simulink library "rocket_angular_flight_library"  (R2014a)
settings: Solver=ode45  StartTime=0.0  StopTime=10.0  RelTol=1e-3
undefined symbols (not defined in the file or in its folder): area_rocket_planform, cog_motor, d_nose_tip_to_fins, d_nose_tip_to_nozzle, diameter_outer, dry_rocket_mass, F, factstruct, fin_center_distance, fin_root_chord, fin_tip_chord, fins_count, height_fins, height_nose_cone, length_motor, Light, mass_flow_rate, MIL, motorburntime
libraries: rocket_angular_flight_library x10, rocket_dynamic_data_library x3, simulink x2, aerolibadyn x2, aerolibbdyn x2, aerolib6dof2 x1, aerolibasang x1, aerolibwind2 x1
settings Model: Creator=scorpii  LastModifiedBy=scorpii

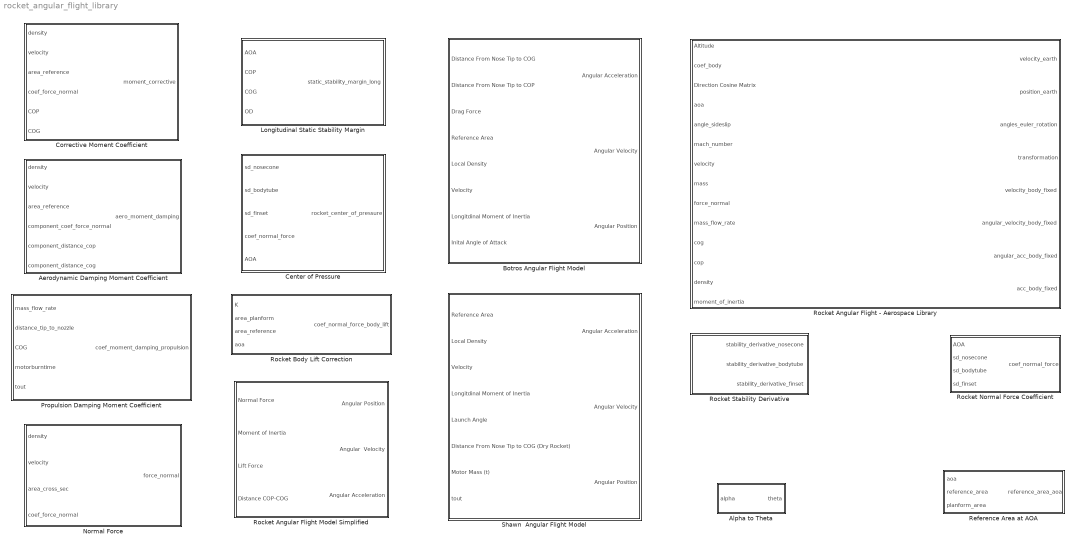
== system rocket_angular_flight_library ==
  Aerodynamic Damping Moment Coefficient : Subsystem  AncestorBlock=rocket_angular_flight_library/Corrective Moment Coefficient
  Alpha to Theta : Subsystem
  Botros Angular Flight Model : Subsystem
  Center of Pressure : Subsystem
  Corrective Moment Coefficient : Subsystem
  Longitudinal Static Stability Margin : Subsystem
  Normal Force : Subsystem
  Propulsion Damping Moment Coefficient : Subsystem
  Reference Area at AOA : Subsystem
  Rocket Angular Flight - Aerospace Library : Subsystem
  Rocket Angular Flight Model Simplified : Subsystem  AncestorBlock=rocket_vertical_flight_library/Rocket Vertical Flight Model
  Rocket Body Lift Correction : Subsystem
  Rocket Normal Force Coefficient : Subsystem
  Rocket Stability Derivative : Subsystem  TreatAsAtomicUnit=on
  Shawn  Angular Flight Model : Subsystem  AncestorBlock=rocket_angular_flight_library/Angular Flight Model

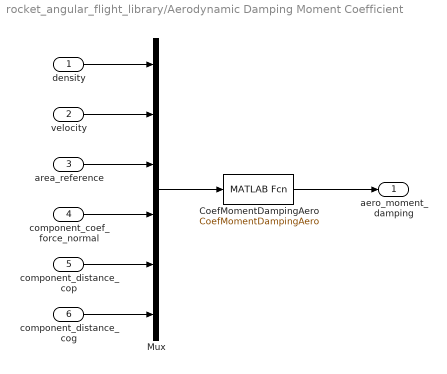
== system rocket_angular_flight_library/Aerodynamic Damping Moment Coefficient ==
  density : Inport
  velocity : Inport  Port=2
  area_reference : Inport  Port=3
  component_coef_force_normal : Inport  Port=4
  component_distance_cop : Inport  Port=5
  component_distance_cog : Inport  Port=6
  CoefMomentDampingAero : MATLABFcn  MATLABFcn=CoefMomentDampingAero
  Mux : Mux  Inputs=6
  aero_moment_damping : Outport
  wires:
  density/1 -> Mux/1
  velocity/1 -> Mux/2
  area_reference/1 -> Mux/3
  component_coef_force_normal/1 -> Mux/4
  component_distance_cop/1 -> Mux/5
  component_distance_cog/1 -> Mux/6
  Mux/1 -> CoefMomentDampingAero/1
  CoefMomentDampingAero/1 -> aero_moment_damping/1

== system rocket_angular_flight_library/Alpha to Theta ==
  alpha : Inport
  Abs : Abs
  Constant : Constant  Value=pi/2
  Subtract : Sum  Inputs=+-
  theta : Outport
  wires:
  Constant/1 -> Subtract/1
  alpha/1 -> Subtract/2
  Subtract/1 -> Abs/1
  Abs/1 -> theta/1

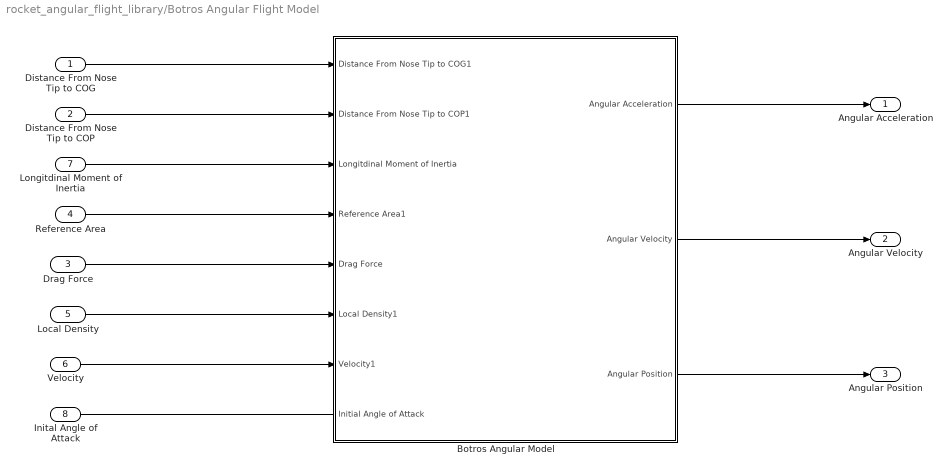
== system rocket_angular_flight_library/Botros Angular Flight Model ==
  Distance From Nose Tip to COG : Inport
  Distance From Nose Tip to COP : Inport  Port=2
  Drag Force : Inport  Port=3
  Reference Area : Inport  Port=4
  Local Density : Inport  Port=5
  Velocity : Inport  Port=6
  "Longitdinal Moment of Inertia " : Inport  Port=7
  Inital Angle of Attack : Inport  Port=8
  Botros Angular Model : Subsystem
  Angular Acceleration : Outport
  Angular Velocity : Outport  Port=2
  Angular Position : Outport  Port=3
  wires:
  Distance From Nose Tip to COP/1 -> Botros Angular Model/2(Distance From Nose Tip to COP1)
  Drag Force/1 -> Botros Angular Model/5(Drag Force)
  Velocity/1 -> Botros Angular Model/7(Velocity1)
  Local Density/1 -> Botros Angular Model/6(Local Density1)
  Reference Area/1 -> Botros Angular Model/4(Reference Area1)
  Botros Angular Model/3(Angular Position) -> Angular Position/1
  Botros Angular Model/1(Angular Acceleration) -> Angular Acceleration/1
  Botros Angular Model/2(Angular Velocity) -> Angular Velocity/1
  "Longitdinal Moment of Inertia "/1 -> Botros Angular Model/3(Longitdinal Moment of Inertia)
  Inital Angle of Attack/1 -> ?
  Distance From Nose Tip to COG/1 -> Botros Angular Model/1(Distance From Nose Tip to COG1)

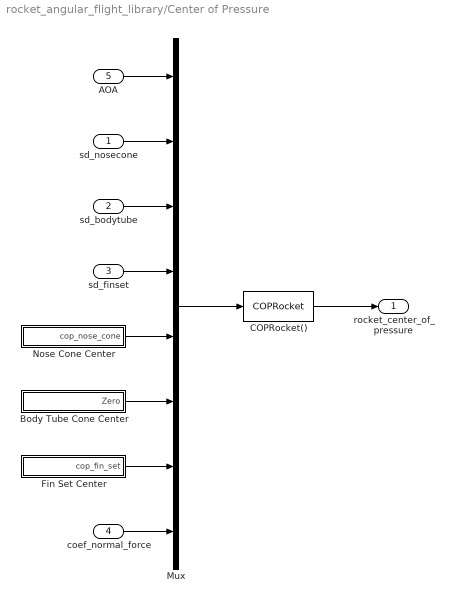
== system rocket_angular_flight_library/Center of Pressure ==
  sd_nosecone : Inport
  sd_bodytube : Inport  Port=2
  sd_finset : Inport  Port=3
  coef_normal_force : Inport  Port=4
  AOA : Inport  Port=5
  Body Tube Cone Center : Subsystem  AncestorBlock=rocket_angular_flight_library/Center of Pressure/Nose Cone Center
  COPRocket() : MATLABFcn  MATLABFcn=COPRocket
  Fin Set Center : Subsystem
  Mux : Mux  Inputs=8
  Nose Cone Center : Subsystem  AncestorBlock=rocket_angular_flight_library/Center of Pressure/Nose Cone Center
  rocket_center_of_pressure : Outport
  wires:
  Mux/1 -> COPRocket()/1
  COPRocket()/1 -> rocket_center_of_pressure/1
  AOA/1 -> Mux/1
  coef_normal_force/1 -> Mux/8
  sd_nosecone/1 -> Mux/2
  sd_bodytube/1 -> Mux/3
  sd_finset/1 -> Mux/4
  Nose Cone Center/1(cop_nose_cone) -> Mux/5
  Fin Set Center/1(cop_fin_set) -> Mux/7
  Body Tube Cone Center/1(Zero) -> Mux/6

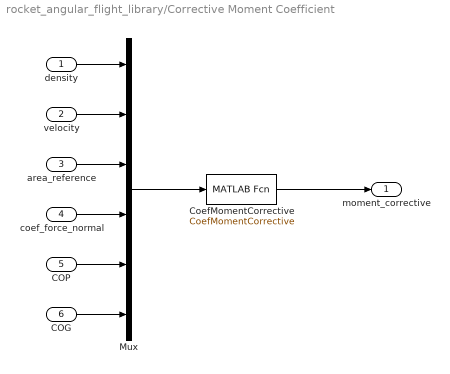
== system rocket_angular_flight_library/Corrective Moment Coefficient ==
  density : Inport
  velocity : Inport  Port=2
  area_reference : Inport  Port=3
  coef_force_normal : Inport  Port=4
  COP : Inport  Port=5
  COG : Inport  Port=6
  CoefMomentCorrective : MATLABFcn  MATLABFcn=CoefMomentCorrective
  Mux : Mux  Inputs=6
  moment_corrective : Outport
  wires:
  density/1 -> Mux/1
  velocity/1 -> Mux/2
  area_reference/1 -> Mux/3
  coef_force_normal/1 -> Mux/4
  COP/1 -> Mux/5
  COG/1 -> Mux/6
  Mux/1 -> CoefMomentCorrective/1
  CoefMomentCorrective/1 -> moment_corrective/1

== system rocket_angular_flight_library/Longitudinal Static Stability Margin ==
  AOA : Inport
  COP : Inport  Port=2
  COG : Inport  Port=3
  OD : Inport  Port=4
  Mux : Mux
  StaticStabilityMarginLong : MATLABFcn  MATLABFcn=StaticStabilityMarginLong
  static_stability_margin_long : Outport
  wires:
  AOA/1 -> Mux/1
  COP/1 -> Mux/2
  COG/1 -> Mux/3
  OD/1 -> Mux/4
  Mux/1 -> StaticStabilityMarginLong/1
  StaticStabilityMarginLong/1 -> static_stability_margin_long/1

== system rocket_angular_flight_library/Normal Force ==
  density : Inport
  velocity : Inport  Port=2
  area_cross_sec : Inport  Port=3
  coef_force_normal : Inport  Port=4
  ForceNormal(inputs) : MATLABFcn  MATLABFcn=ForceNormal
  Mux : Mux
  force_normal : Outport
  wires:
  density/1 -> Mux/1
  velocity/1 -> Mux/2
  area_cross_sec/1 -> Mux/3
  coef_force_normal/1 -> Mux/4
  Mux/1 -> ForceNormal(inputs)/1
  ForceNormal(inputs)/1 -> force_normal/1

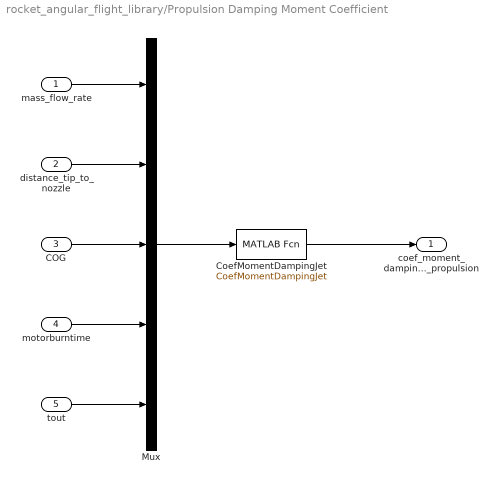
== system rocket_angular_flight_library/Propulsion Damping Moment Coefficient ==
  mass_flow_rate : Inport
  distance_tip_to_nozzle : Inport  Port=2
  COG : Inport  Port=3
  motorburntime : Inport  Port=4
  tout : Inport  Port=5
  CoefMomentDampingJet : MATLABFcn  MATLABFcn=CoefMomentDampingJet
  Mux : Mux  Inputs=5
  coef_moment_damping_propulsion : Outport
  wires:
  Mux/1 -> CoefMomentDampingJet/1
  mass_flow_rate/1 -> Mux/1
  distance_tip_to_nozzle/1 -> Mux/2
  COG/1 -> Mux/3
  CoefMomentDampingJet/1 -> coef_moment_damping_propulsion/1
  motorburntime/1 -> Mux/4
  tout/1 -> Mux/5

== system rocket_angular_flight_library/Reference Area at AOA ==
  aoa : Inport
  reference_area : Inport  Port=2
  planform_area : Inport  Port=3
  reference_area_aoa : Outport
  wires:
  reference_area/1 -> reference_area_aoa/1

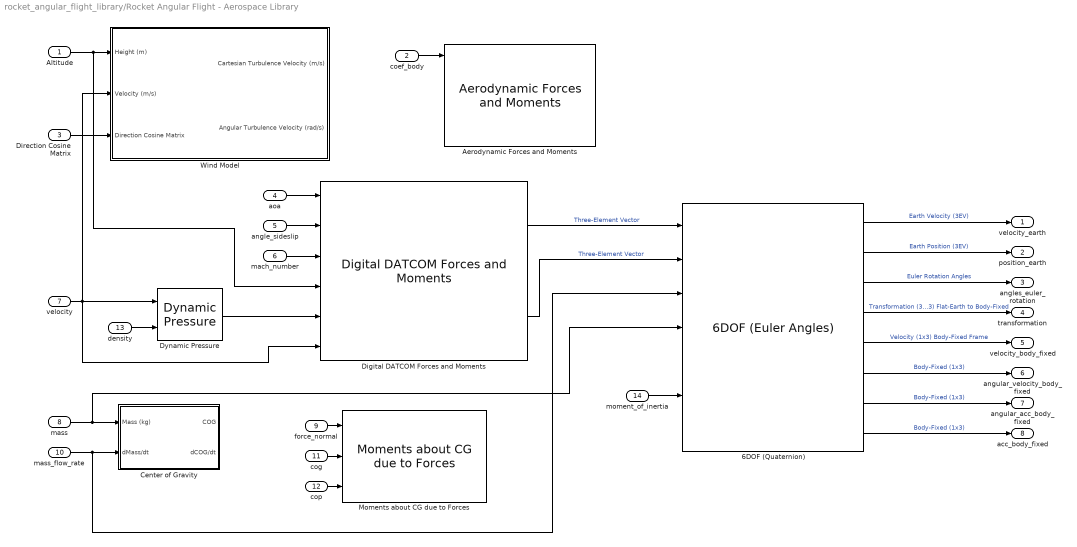
== system rocket_angular_flight_library/Rocket Angular Flight - Aerospace Library ==
  Altitude : Inport
  coef_body : Inport  Port=2
  Direction Cosine Matrix : Inport  Port=3
  aoa : Inport  Port=4
  angle_sideslip : Inport  Port=5
  mach_number : Inport  Port=6
  velocity : Inport  Port=7
  mass : Inport  Port=8
  force_normal : Inport  Port=9
  mass_flow_rate : Inport  Port=10
  cog : Inport  Port=11
  cop : Inport  Port=12
  density : Inport  Port=13
  moment_of_inertia : Inport  Port=14
  6DOF (Quaternion) : aerolib6dof2/6DOF (Euler Angles)  units=Metric (MKS)  mtype=Custom Variable  rep=Quaternion  xme_0=[0 0 0]  Vm_0=[0 0 0]  eul_0=[0 0 0]  pm_0=[0 0 0]  mass_0=1.0  mass_e=0.5  mass_f=2.0  inertia=eye(3)  inertia_e=eye(3)  inertia_f=2*eye(3)  k_quat=1.0  vre_flag=on
  "Aerodynamic Forces and Moments " : aerolibadyn/Aerodynamic Forces and Moments   inputAxes=Body  outputForceAxes=Body  outputMomentAxes=Body  S=1  b=1  cbar=1
  Center of Gravity : Subsystem
  Digital DATCOM Forces and Moments : aerolibadyn/Digital DATCOM Forces and Moments  units=Metric (MKS)  dcase=factstruct{1}  fmode=Body  buildno=0  imethod=Linear  emethod=Linear  rmethod=Linear Extrapolation  action=None
  Dynamic Pressure : aerolibasang/Dynamic Pressure
  Moments about CG due to Forces : aerolibbdyn/Moments about CG  due to Forces
  Wind Model : Subsystem
  velocity_earth : Outport
  position_earth : Outport  Port=2
  angles_euler_rotation : Outport  Port=3
  transformation : Outport  Port=4
  velocity_body_fixed : Outport  Port=5
  angular_velocity_body_fixed : Outport  Port=6
  angular_acc_body_fixed : Outport  Port=7
  acc_body_fixed : Outport  Port=8
  wires:
  cog/1 -> Moments about CG due to Forces/2
  coef_body/1 -> "Aerodynamic Forces and Moments "/1
  cop/1 -> Moments about CG due to Forces/3
  6DOF (Quaternion)/1 -> velocity_earth/1  "Earth Velocity (3EV)"
  density/1 -> Dynamic Pressure/2
  Direction Cosine Matrix/1 -> Wind Model/3(Direction Cosine Matrix)
  force_normal/1 -> Moments about CG due to Forces/1
  6DOF (Quaternion)/8 -> acc_body_fixed/1  "Body-Fixed (1x3)"
  6DOF (Quaternion)/6 -> angular_velocity_body_fixed/1  "Body-Fixed (1x3)"
  6DOF (Quaternion)/7 -> angular_acc_body_fixed/1  "Body-Fixed (1x3)"
  6DOF (Quaternion)/2 -> position_earth/1  "Earth Position (3EV)"
  6DOF (Quaternion)/3 -> angles_euler_rotation/1  "Euler Rotation Angles"
  velocity/1 -> Digital DATCOM Forces and Moments/6, Wind Model/2(Velocity (m/s)), Dynamic Pressure/1
  6DOF (Quaternion)/4 -> transformation/1  "Transformation (3x3) Flat-Earth to Body-Fixed"
  6DOF (Quaternion)/5 -> velocity_body_fixed/1  "Velocity (1x3) Body-Fixed Frame"
  mass/1 -> 6DOF (Quaternion)/4, Center of Gravity/1(Mass (kg))
  aoa/1 -> Digital DATCOM Forces and Moments/1
  angle_sideslip/1 -> Digital DATCOM Forces and Moments/2
  mass_flow_rate/1 -> 6DOF (Quaternion)/3, Center of Gravity/2(dMass/dt)
  mach_number/1 -> Digital DATCOM Forces and Moments/3
  Dynamic Pressure/1 -> Digital DATCOM Forces and Moments/5
  Digital DATCOM Forces and Moments/1 -> 6DOF (Quaternion)/1  "Three-Element Vector"
  Digital DATCOM Forces and Moments/2 -> 6DOF (Quaternion)/2  "Three-Element Vector"
  Altitude/1 -> Digital DATCOM Forces and Moments/4, Wind Model/1(Height (m))
  moment_of_inertia/1 -> 6DOF (Quaternion)/6

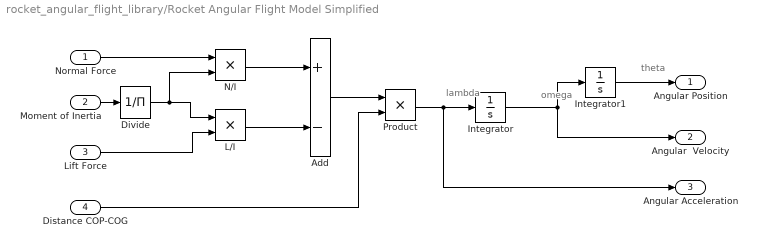
== system rocket_angular_flight_library/Rocket Angular Flight Model Simplified ==
  note: lambda
  note: theta
  note: omega
  Normal Force : Inport
  Moment of Inertia : Inport  Port=2
  Lift Force : Inport  Port=3
  Distance COP-COG : Inport  Port=4
  Add : Sum  Inputs=+-
  Divide : Product  Inputs=/
  Integrator : Integrator
  Integrator1 : Integrator
  L/I : Product
  N/I : Product
  Product : Product
  Angular Position : Outport
  Angular  Velocity : Outport  Port=2
  Angular Acceleration : Outport  Port=3
  wires:
  Divide/1 -> L/I/1, N/I/2
  L/I/1 -> Add/2
  N/I/1 -> Add/1
  Integrator/1 -> Integrator1/1, Angular  Velocity/1
  Integrator1/1 -> Angular Position/1
  Lift Force/1 -> L/I/2
  Moment of Inertia/1 -> Divide/1
  Normal Force/1 -> N/I/1
  Add/1 -> Product/1
  Product/1 -> Angular Acceleration/1, Integrator/1
  Distance COP-COG/1 -> Product/2

== system rocket_angular_flight_library/Rocket Body Lift Correction ==
  K : Inport
  area_planform : Inport  Port=2
  area_reference : Inport  Port=3
  aoa : Inport  Port=4
  CoefNormalForceBodyLift : MATLABFcn  MATLABFcn=CoefNormalForceBodyLift
  Mux : Mux
  coef_normal_force_body_lift : Outport
  wires:
  K/1 -> Mux/1
  area_planform/1 -> Mux/2
  area_reference/1 -> Mux/3
  Mux/1 -> CoefNormalForceBodyLift/1
  CoefNormalForceBodyLift/1 -> coef_normal_force_body_lift/1
  aoa/1 -> Mux/4

== system rocket_angular_flight_library/Rocket Normal Force Coefficient ==
  AOA : Inport
  sd_nosecone : Inport  Port=2
  sd_bodytube : Inport  Port=3
  sd_finset : Inport  Port=4
  Add1 : Sum  Inputs=+++
  Product : Product
  Small Angle Approximation : Subsystem
  coef_normal_force : Outport
  wires:
  AOA/1 -> Small Angle Approximation/1(Angle)
  sd_nosecone/1 -> Add1/1
  sd_bodytube/1 -> Add1/2
  sd_finset/1 -> Add1/3
  Add1/1 -> Product/2
  Small Angle Approximation/1(Out) -> Product/1
  Product/1 -> coef_normal_force/1

== system rocket_angular_flight_library/Rocket Stability Derivative ==
  Body Tube Stability Derivative : Subsystem
  Fin Set Stability Derivative : Subsystem
  Nose Cone Stability Derivative : Subsystem
  stability_derivative_nosecone : Outport
  stability_derivative_bodytube : Outport  Port=2
  stability_derivative_finset : Outport  Port=3
  wires:
  Nose Cone Stability Derivative/1(Two) -> stability_derivative_nosecone/1
  Body Tube Stability Derivative/1(Zero) -> stability_derivative_bodytube/1
  Fin Set Stability Derivative/1(stability_derivative_fin_set) -> stability_derivative_finset/1

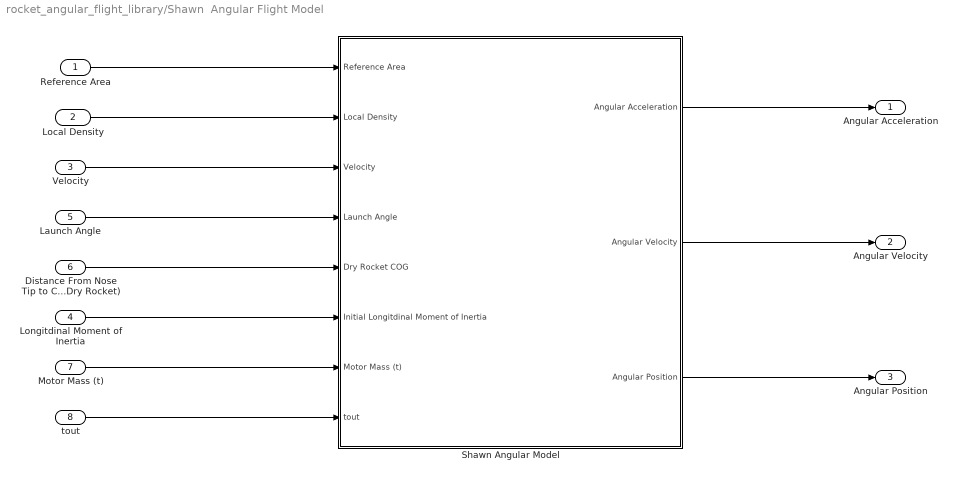
== system rocket_angular_flight_library/Shawn  Angular Flight Model ==
  Reference Area : Inport
  Local Density : Inport  Port=2
  Velocity : Inport  Port=3
  "Longitdinal Moment of Inertia " : Inport  Port=4
  Launch Angle : Inport  Port=5
  Distance From Nose Tip to COG (Dry Rocket) : Inport  Port=6
  Motor Mass (t) : Inport  Port=7
  tout : Inport  Port=8
  Shawn Angular Model : Subsystem
  Angular Acceleration : Outport
  Angular Velocity : Outport  Port=2
  Angular Position : Outport  Port=3
  wires:
  Velocity/1 -> Shawn Angular Model/3(Velocity)
  Local Density/1 -> Shawn Angular Model/2(Local Density)
  Reference Area/1 -> Shawn Angular Model/1(Reference Area)
  Shawn Angular Model/3(Angular Position) -> Angular Position/1
  Shawn Angular Model/1(Angular Acceleration) -> Angular Acceleration/1
  Shawn Angular Model/2(Angular Velocity) -> Angular Velocity/1
  Launch Angle/1 -> Shawn Angular Model/4(Launch Angle)
  Distance From Nose Tip to COG (Dry Rocket)/1 -> Shawn Angular Model/5(Dry Rocket COG)
  "Longitdinal Moment of Inertia "/1 -> Shawn Angular Model/6(Initial Longitdinal Moment of Inertia)
  Motor Mass (t)/1 -> Shawn Angular Model/7(Motor Mass (t))
  tout/1 -> Shawn Angular Model/8(tout)

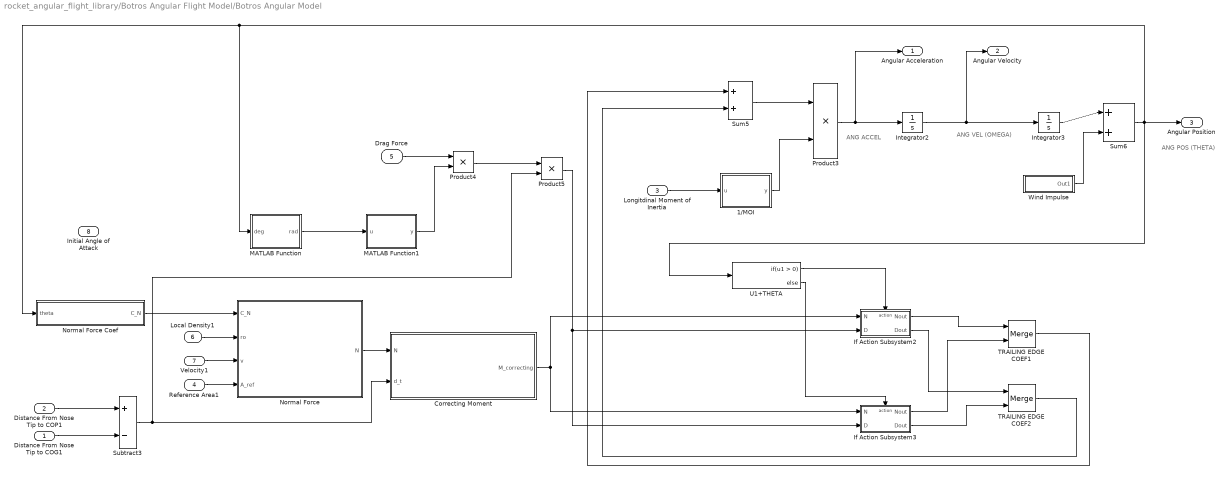
== system rocket_angular_flight_library/Botros Angular Flight Model/Botros Angular Model ==
  note: ANG ACCEL
  note: ANG POS (THETA)
  note: ANG VEL (OMEGA)
  Distance From Nose Tip to COG1 : Inport
  Distance From Nose Tip to COP1 : Inport  Port=2
  Longitdinal Moment of Inertia : Inport  Port=3
  Reference Area1 : Inport  Port=4
  Drag Force : Inport  Port=5
  Local Density1 : Inport  Port=6
  Velocity1 : Inport  Port=7
  Initial Angle of Attack : Inport  Port=8
  1/MOI : Subsystem  TreatAsAtomicUnit=on
  Correcting Moment : Subsystem  TreatAsAtomicUnit=on
  If Action Subsystem2 : Subsystem  TreatAsAtomicUnit=on
  If Action Subsystem3 : Subsystem  TreatAsAtomicUnit=on
  Integrator2 : Integrator
  Integrator3 : Integrator
  MATLAB Function : Subsystem  TreatAsAtomicUnit=on
  MATLAB Function1 : Subsystem  TreatAsAtomicUnit=on
  Normal Force : Subsystem  TreatAsAtomicUnit=on
  Normal Force Coef : Subsystem  TreatAsAtomicUnit=on
  Product3 : Product
  Product4 : Product
  Product5 : Product
  Subtract3 : Sum  Inputs=+-
  Sum5 : Sum
  Sum6 : Sum  Inputs=|++
  TRAILING EDGE COEF1 : Merge
  TRAILING EDGE COEF2 : Merge
  U1+THETA : If
  Wind Impulse : Subsystem
  Angular Acceleration : Outport
  Angular Velocity : Outport  Port=2
  Angular Position : Outport  Port=3
  wires:
  If Action Subsystem2/2(Dout) -> TRAILING EDGE COEF2/1
  Normal Force Coef/1(C_N) -> Normal Force/1(C_N)
  Sum6/1 -> Angular Position/1, MATLAB Function/1(deg), Normal Force Coef/1(theta), U1+THETA/1
  Velocity1/1 -> Normal Force/3(v)
  Distance From Nose Tip to COP1/1 -> Subtract3/1
  Product3/1 -> Integrator2/1, Angular Acceleration/1
  Integrator3/1 -> Sum6/1
  TRAILING EDGE COEF1/1 -> Sum5/1
  TRAILING EDGE COEF2/1 -> Sum5/2
  Distance From Nose Tip to COG1/1 -> Subtract3/2
  MATLAB Function1/1(y) -> Product4/2
  Local Density1/1 -> Normal Force/2(ro)
  Sum5/1 -> Product3/1
  MATLAB Function/1(rad) -> MATLAB Function1/1(u)
  U1+THETA/1 -> If Action Subsystem2/Action
  Normal Force/1(N) -> Correcting Moment/1(N)
  U1+THETA/2 -> If Action Subsystem3/Action
  Product4/1 -> Product5/1
  If Action Subsystem2/1(Nout) -> TRAILING EDGE COEF1/1
  If Action Subsystem3/2(Dout) -> TRAILING EDGE COEF2/2
  Correcting Moment/1(M_correcting) -> If Action Subsystem2/1(N), If Action Subsystem3/1(N)
  1/MOI/1(y) -> Product3/2
  Reference Area1/1 -> Normal Force/4(A_ref)
  Integrator2/1 -> Integrator3/1, Angular Velocity/1
  Product5/1 -> If Action Subsystem3/2(D), If Action Subsystem2/2(D)
  Subtract3/1 -> Product5/2, Correcting Moment/2(d_t)
  If Action Subsystem3/1(Nout) -> TRAILING EDGE COEF1/2
  Drag Force/1 -> Product4/1
  Wind Impulse/1(Out1) -> Sum6/2
  Longitdinal Moment of Inertia/1 -> 1/MOI/1(u)

== system rocket_angular_flight_library/Center of Pressure/Body Tube Cone Center ==
  Assume Zero Body Lift : Constant  Value=0
  Zero : Outport
  wires:
  Assume Zero Body Lift/1 -> Zero/1

== system rocket_angular_flight_library/Center of Pressure/Fin Set Center ==
  Distance from nose tip to fins at base : Constant  Value=d_nose_tip_to_fins
  Fin Center Distance : Constant  Value=fin_center_distance
  "Fin Root Chord " : Constant  Value=fin_root_chord
  Fin Set COP : MATLABFcn  MATLABFcn=COPFinSet
  Fin Tip Chord : Constant  Value=fin_tip_chord
  Mux : Mux
  cop_fin_set : Outport
  wires:
  Fin Center Distance/1 -> Mux/1
  "Fin Root Chord "/1 -> Mux/2
  Fin Tip Chord/1 -> Mux/3
  Mux/1 -> Fin Set COP/1
  Fin Set COP/1 -> cop_fin_set/1
  Distance from nose tip to fins at base/1 -> Mux/4

== system rocket_angular_flight_library/Center of Pressure/Nose Cone Center ==
  Nose Cone Height : Constant  Value=height_nose_cone
  Von Karman Nose Cone Center of Pressure : MATLABFcn  MATLABFcn=COPNoseConeVonKarman
  cop_nose_cone : Outport
  wires:
  Nose Cone Height/1 -> Von Karman Nose Cone Center of Pressure/1
  Von Karman Nose Cone Center of Pressure/1 -> cop_nose_cone/1

== system rocket_angular_flight_library/Rocket Angular Flight - Aerospace Library/Center of Gravity ==
  Mass (kg) : Inport
  dMass/dt : Inport  Port=2
  Dynamic Center Of Gravity : rocket_dynamic_data_library/Dynamic Center Of Gravity
  Estimate Center of Gravity : aerolibbdyn/Estimate Center of Gravity  fmass=2  emass=1  fcg=[1 1 1]'  ecg=[0.5 0.5 0.5]'
  COG : Outport
  dCOG/dt : Outport  Port=2
  wires:
  Mass (kg)/1 -> COG/1
  dMass/dt/1 -> dCOG/dt/1

== system rocket_angular_flight_library/Rocket Angular Flight - Aerospace Library/Wind Model ==
  Height (m) : Inport
  Velocity (m/s) : Inport  Port=2
  Direction Cosine Matrix : Inport  Port=3
  Von Karman Wind Turbulence Model (Continuous (+q +r)) : aerolibwind2/Dryden Wind Turbulence Model  (Continuous (+q -r))  units=Metric (MKS)  spec=MIL-F-8785C  model=Continuous Von Karman (+q +r)  W20=15  Wdeg=0  TurbProb=10^-2 - Light  L_high=762  Wingspan=10  ts=0.1  Seed=[23341 23342 23343 23344]  T_on=on
  Cartesian Turbulence Velocity (m/s) : Outport
  Angular Turbulence Velocity (rad/s) : Outport  Port=2
  wires:
  Von Karman Wind Turbulence Model (Continuous (+q +r))/2 -> Angular Turbulence Velocity (rad/s)/1
  Von Karman Wind Turbulence Model (Continuous (+q +r))/1 -> Cartesian Turbulence Velocity (m/s)/1
  Height (m)/1 -> Von Karman Wind Turbulence Model (Continuous (+q +r))/1
  Velocity (m/s)/1 -> Von Karman Wind Turbulence Model (Continuous (+q +r))/2
  Direction Cosine Matrix/1 -> Von Karman Wind Turbulence Model (Continuous (+q +r))/3

== system rocket_angular_flight_library/Rocket Normal Force Coefficient/Small Angle Approximation ==
  Angle : Inport
  Out : Outport
  wires:
  Angle/1 -> Out/1

== system rocket_angular_flight_library/Rocket Stability Derivative/Body Tube Stability Derivative ==
  Assume Zero Body Lift : Constant  Value=0
  Zero : Outport
  wires:
  Assume Zero Body Lift/1 -> Zero/1

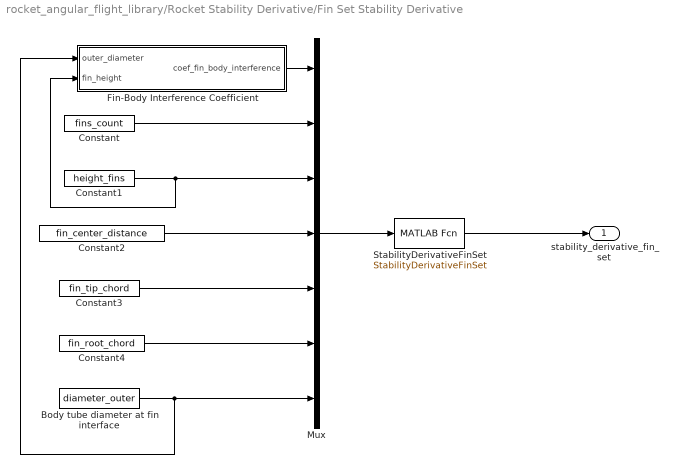
== system rocket_angular_flight_library/Rocket Stability Derivative/Fin Set Stability Derivative ==
  Body tube diameter at fin interface : Constant  Value=diameter_outer
  Constant : Constant  Value=fins_count
  Constant1 : Constant  Value=height_fins
  Constant2 : Constant  Value=fin_center_distance
  Constant3 : Constant  Value=fin_tip_chord
  Constant4 : Constant  Value=fin_root_chord
  Fin-Body Interference Coefficient : Subsystem
  Mux : Mux  Inputs=7
  StabilityDerivativeFinSet : MATLABFcn  MATLABFcn=StabilityDerivativeFinSet
  stability_derivative_fin_set : Outport
  wires:
  Mux/1 -> StabilityDerivativeFinSet/1
  Constant/1 -> Mux/2
  Constant1/1 -> Fin-Body Interference Coefficient/2(fin_height), Mux/3
  Constant2/1 -> Mux/4
  Constant3/1 -> Mux/5
  Constant4/1 -> Mux/6
  Body tube diameter at fin interface/1 -> Fin-Body Interference Coefficient/1(outer_diameter), Mux/7
  Fin-Body Interference Coefficient/1(coef_fin_body_interference) -> Mux/1
  StabilityDerivativeFinSet/1 -> stability_derivative_fin_set/1

== system rocket_angular_flight_library/Rocket Stability Derivative/Nose Cone Stability Derivative ==
  "Asummed for: Ogive, Parabolic, Conical" : Constant  Value=2
  Two : Outport
  wires:
  "Asummed for: Ogive, Parabolic, Conical"/1 -> Two/1

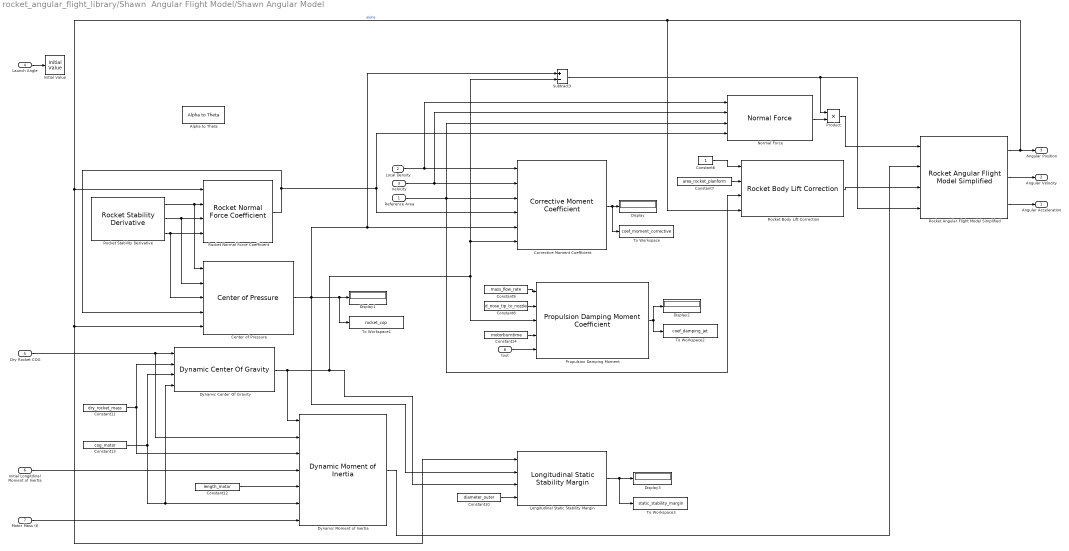
== system rocket_angular_flight_library/Shawn  Angular Flight Model/Shawn Angular Model ==
  Reference Area : Inport
  Local Density : Inport  Port=2
  Velocity : Inport  Port=3
  Launch Angle : Inport  Port=4
  Dry Rocket COG : Inport  Port=5
  Initial Longitdinal Moment of Inertia : Inport  Port=6
  Motor Mass (t) : Inport  Port=7
  tout : Inport  Port=8
  Alpha to Theta : rocket_angular_flight_library/Alpha to Theta
  Center of Pressure : rocket_angular_flight_library/Center of Pressure
  Constant10 : Constant  Value=diameter_outer
  Constant11 : Constant  Value=dry_rocket_mass
  Constant12 : Constant  Value=length_motor
  Constant13 : Constant  Value=cog_motor
  Constant14 : Constant  Value=motorburntime
  Constant6 : Constant
  Constant7 : Constant  Value=area_rocket_planform
  Constant8 : Constant  Value=d_nose_tip_to_nozzle
  Constant9 : Constant  Value=mass_flow_rate
  Corrective Moment Coefficient : rocket_angular_flight_library/Corrective Moment Coefficient
  Display{,1..3} (4 alike) : Display
  Dynamic Center Of Gravity : rocket_dynamic_data_library/Dynamic Center Of Gravity
  Dynamic Moment of Inertia : rocket_dynamic_data_library/Dynamic Moment of Inertia
  Initial Value : InitialValue  InitialValue=launch_angle
  Longitudinal Static Stability Margin : rocket_angular_flight_library/Longitudinal Static Stability Margin  SystemSampleTime=-1
  Normal Force : rocket_angular_flight_library/Normal Force
  Product : Product
  Propulsion Damping Moment : rocket_angular_flight_library/Propulsion Damping Moment Coefficient  SystemSampleTime=-1
  Rocket Angular Flight Model Simplified : rocket_angular_flight_library/Rocket Angular Flight Model Simplified
  Rocket Body Lift Correction : rocket_angular_flight_library/Rocket Body Lift Correction
  Rocket Normal Force Coefficient : rocket_angular_flight_library/Rocket Normal Force Coefficient
  Rocket Stability Derivative : rocket_angular_flight_library/Rocket Stability Derivative
  Subtract3 : Sum  Inputs=+-
  To Workspace : ToWorkspace  VariableName=coef_moment_corrective  SaveFormat=Timeseries  SampleTime=-1
  To Workspace1 : ToWorkspace  VariableName=rocket_cop  SaveFormat=Timeseries  SampleTime=-1
  To Workspace2 : ToWorkspace  VariableName=coef_damping_jet  SaveFormat=Timeseries  SampleTime=-1
  To Workspace3 : ToWorkspace  VariableName=static_stability_margin  SaveFormat=Timeseries  SampleTime=-1
  Angular Acceleration : Outport
  Angular Velocity : Outport  Port=2
  Angular Position : Outport  Port=3
  wires:
  Rocket Angular Flight Model Simplified/1 -> Rocket Normal Force Coefficient/1, Center of Pressure/5, Longitudinal Static Stability Margin/1, Rocket Body Lift Correction/4, Angular Position/1  "alpha"
  Subtract3/1 -> Rocket Angular Flight Model Simplified/4, Product/1
  Product/1 -> Rocket Angular Flight Model Simplified/1
  Rocket Angular Flight Model Simplified/2 -> Angular Velocity/1
  Rocket Angular Flight Model Simplified/3 -> Angular Acceleration/1
  Launch Angle/1 -> Initial Value/1
  Local Density/1 -> Normal Force/1, Corrective Moment Coefficient/1
  Velocity/1 -> Corrective Moment Coefficient/2, Normal Force/2
  Rocket Normal Force Coefficient/1 -> Corrective Moment Coefficient/4, Normal Force/4, Center of Pressure/4
  Dynamic Center Of Gravity/1 -> Dynamic Moment of Inertia/1, Corrective Moment Coefficient/6, Subtract3/2, Propulsion Damping Moment/3, Longitudinal Static Stability Margin/3
  Rocket Body Lift Correction/1 -> Rocket Angular Flight Model Simplified/3
  Constant6/1 -> Rocket Body Lift Correction/1
  Constant7/1 -> Rocket Body Lift Correction/2
  Reference Area/1 -> Corrective Moment Coefficient/3, Normal Force/3, Rocket Body Lift Correction/3
  Constant8/1 -> Propulsion Damping Moment/2
  Constant9/1 -> Propulsion Damping Moment/1
  Normal Force/1 -> Product/2
  Corrective Moment Coefficient/1 -> To Workspace/1, Display/1
  Propulsion Damping Moment/1 -> Display2/1, To Workspace2/1
  Rocket Stability Derivative/1 -> Center of Pressure/1, Rocket Normal Force Coefficient/2
  Rocket Stability Derivative/2 -> Center of Pressure/2, Rocket Normal Force Coefficient/3
  Rocket Stability Derivative/3 -> Center of Pressure/3, Rocket Normal Force Coefficient/4
  Dry Rocket COG/1 -> Dynamic Center Of Gravity/1, Dynamic Moment of Inertia/2
  Initial Longitdinal Moment of Inertia/1 -> Dynamic Moment of Inertia/4
  Constant10/1 -> Longitudinal Static Stability Margin/4
  Longitudinal Static Stability Margin/1 -> To Workspace3/1, Display3/1
  Constant11/1 -> Dynamic Moment of Inertia/3, Dynamic Center Of Gravity/2
  Constant12/1 -> Dynamic Moment of Inertia/5
  Constant13/1 -> Dynamic Center Of Gravity/4, Dynamic Moment of Inertia/6, Dynamic Center Of Gravity/3
  tout/1 -> Propulsion Damping Moment/5
  Motor Mass (t)/1 -> Dynamic Moment of Inertia/7
  Constant14/1 -> Propulsion Damping Moment/4
  Dynamic Moment of Inertia/1 -> Rocket Angular Flight Model Simplified/2
  Center of Pressure/1 -> To Workspace1/1, Display1/1, Longitudinal Static Stability Margin/2, Subtract3/1, Corrective Moment Coefficient/5

== system rocket_angular_flight_library/Botros Angular Flight Model/Botros Angular Model/1//MOI ==
  u : Inport
  " Demux " : Demux  Outputs=1
  " SFunction " : S-Function  Tag=Stateflow S-Function VELOCITY_MODEL 37  FunctionName=sf_sfun  PortCounts=[1 2]  EnableBusSupport=on
  " Terminator " : Terminator
  y : Outport
  wires:
  u/1 -> " SFunction "/1
  " SFunction "/2 -> y/1  "y"
  " Demux "/1 -> " Terminator "/1
  " SFunction "/1 -> " Demux "/1

== system rocket_angular_flight_library/Botros Angular Flight Model/Botros Angular Model/Correcting Moment ==
  N : Inport
  d_t : Inport  Port=2
  " Demux " : Demux  Outputs=1
  " SFunction " : S-Function  Tag=Stateflow S-Function VELOCITY_MODEL 34  FunctionName=sf_sfun  PortCounts=[2 2]  EnableBusSupport=on
  " Terminator " : Terminator
  M_correcting : Outport
  wires:
  N/1 -> " SFunction "/1
  d_t/1 -> " SFunction "/2
  " SFunction "/2 -> M_correcting/1  "M_correcting"
  " Demux "/1 -> " Terminator "/1
  " SFunction "/1 -> " Demux "/1

== system rocket_angular_flight_library/Botros Angular Flight Model/Botros Angular Model/If Action Subsystem2 ==
  N : Inport
  D : Inport  Port=2
  Action Port : ActionPort
  Gain : Gain  Gain=-1
  Gain1 : Gain  Gain=-1
  Nout : Outport
  Dout : Outport  Port=2
  wires:
  N/1 -> Gain/1
  Gain/1 -> Nout/1
  D/1 -> Gain1/1
  Gain1/1 -> Dout/1

== system rocket_angular_flight_library/Botros Angular Flight Model/Botros Angular Model/If Action Subsystem3 ==
  N : Inport
  D : Inport  Port=2
  Action Port : ActionPort
  Gain : Gain
  Gain1 : Gain
  Nout : Outport
  Dout : Outport  Port=2
  wires:
  N/1 -> Gain/1
  Gain/1 -> Nout/1
  D/1 -> Gain1/1
  Gain1/1 -> Dout/1

== system rocket_angular_flight_library/Botros Angular Flight Model/Botros Angular Model/MATLAB Function ==
  deg : Inport
  " Demux " : Demux  Outputs=1
  " SFunction " : S-Function  Tag=Stateflow S-Function VELOCITY_MODEL 30  FunctionName=sf_sfun  PortCounts=[1 2]  EnableBusSupport=on
  " Terminator " : Terminator
  rad : Outport
  wires:
  deg/1 -> " SFunction "/1
  " SFunction "/2 -> rad/1  "rad"
  " Demux "/1 -> " Terminator "/1
  " SFunction "/1 -> " Demux "/1

== system rocket_angular_flight_library/Botros Angular Flight Model/Botros Angular Model/MATLAB Function1 ==
  u : Inport
  " Demux " : Demux  Outputs=1
  " SFunction " : S-Function  Tag=Stateflow S-Function VELOCITY_MODEL 31  FunctionName=sf_sfun  PortCounts=[1 2]  EnableBusSupport=on
  " Terminator " : Terminator
  y : Outport
  wires:
  u/1 -> " SFunction "/1
  " SFunction "/2 -> y/1  "y"
  " Demux "/1 -> " Terminator "/1
  " SFunction "/1 -> " Demux "/1

== system rocket_angular_flight_library/Botros Angular Flight Model/Botros Angular Model/Normal Force ==
  C_N : Inport
  ro : Inport  Port=2
  v : Inport  Port=3
  A_ref : Inport  Port=4
  " Demux " : Demux  Outputs=1
  " SFunction " : S-Function  Tag=Stateflow S-Function VELOCITY_MODEL 35  FunctionName=sf_sfun  PortCounts=[4 2]  EnableBusSupport=on
  " Terminator " : Terminator
  N : Outport
  wires:
  C_N/1 -> " SFunction "/1
  ro/1 -> " SFunction "/2
  v/1 -> " SFunction "/3
  A_ref/1 -> " SFunction "/4
  " SFunction "/2 -> N/1  "N"
  " Demux "/1 -> " Terminator "/1
  " SFunction "/1 -> " Demux "/1

== system rocket_angular_flight_library/Botros Angular Flight Model/Botros Angular Model/Normal Force Coef ==
  theta : Inport
  " Demux " : Demux  Outputs=1
  " SFunction " : S-Function  Tag=Stateflow S-Function VELOCITY_MODEL 36  FunctionName=sf_sfun  PortCounts=[1 2]  EnableBusSupport=on
  " Terminator " : Terminator
  C_N : Outport
  wires:
  theta/1 -> " SFunction "/1
  " SFunction "/2 -> C_N/1  "C_N"
  " Demux "/1 -> " Terminator "/1
  " SFunction "/1 -> " Demux "/1

== system rocket_angular_flight_library/Botros Angular Flight Model/Botros Angular Model/Wind Impulse ==
  note: WIND IMPULSE
  Gain2 : Gain  Gain=0
  Ramp : simulink/Sources/Ramp  slope=5  start=2  X0=0
  Ramp1 : simulink/Sources/Ramp  slope=-5  start=2.0001  X0=0
  Sum7 : Sum  Inputs=+-
  Out1 : Outport
  wires:
  Gain2/1 -> Out1/1
  Ramp/1 -> Sum7/1
  Ramp1/1 -> Sum7/2
  Sum7/1 -> Gain2/1

== system rocket_angular_flight_library/Rocket Stability Derivative/Fin Set Stability Derivative/Fin-Body Interference Coefficient ==
  outer_diameter : Inport
  fin_height : Inport  Port=2
  Interpreted MATLAB Function : MATLABFcn
  Mux : Mux  Inputs=2
  coef_fin_body_interference : Outport
  wires:
  Interpreted MATLAB Function/1 -> coef_fin_body_interference/1
  Mux/1 -> Interpreted MATLAB Function/1
  outer_diameter/1 -> Mux/1
  fin_height/1 -> Mux/2
